simulink model "BusCreator"  (R2018b)
settings: Solver=FixedStepDiscrete  StartTime=0.0  StopTime=10.0  RelTol=1e-3
settings Model: Creator=mostafa  LastModifiedBy=mostafa
settings DataIOCC: ReturnWorkspaceOutputs=on
settings OptimizationCC: DefaultParameterBehavior=Inlined  EnhancedBackFolding=on  PassReuseOutputArgsAs=Individual arguments  ZeroExternalMemoryAtStartup=off  ZeroInternalMemoryAtStartup=off  OptimizeBlockOrder=speed  DifferentSizesBufferReuse=on  OptimizationCustomize=off
settings DebuggingCC: UnderspecifiedInitializationDetection=Classic  MergeDetectMultiDrivingBlocksExec=none  ParameterTunabilityLossMsg=error  SFMachineParentedDataDiag=error
settings ModelReferenceCC: PropagateSignalLabelsOutOfModel=off
settings SFSimCC: SimCustomHeaderCode="#include \"Interface.h\""  SimUserSources=Interface.h  MATLABDynamicMemAlloc=off
settings RTWCC: SystemTargetFile=ert.tlc  GenCodeOnly=on  TemplateMakefile=ert_default_tmf  GenerateReport=on  IncludeHyperlinkInReport=on  LaunchReport=on  GenerateTraceInfo=on  GenerateTraceReport=on  GenerateTraceReportSl=on  GenerateTraceReportSf=on  GenerateTraceReportEml=on
settings CodeAppCC: ForceParamTrailComments=on  IgnoreCustomStorageClasses=off  OperatorAnnotations=on  SimulinkDataObjDesc=on  SFDataObjDesc=on  InsertBlockDesc=on
settings ERTTargetCC: TargetLangStandard=C99 (ISO)  GenerateSampleERTMain=on  InlinedParameterPlacement=NonHierarchical  ERTCustomFileTemplate=example_file_process.tlc

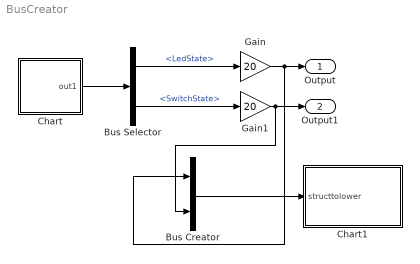
== system BusCreator ==
  Bus Creator : BusCreator  Inputs=2
  Bus Selector : BusSelector  OutputSignals=LedState,SwitchState
  Chart : Stateflow chart  TreatAsAtomicUnit=on
  Chart1 : Stateflow chart  TreatAsAtomicUnit=on
  Gain : Gain  Gain=20
  Gain1 : Gain  Gain=20
  Output : Outport
  Output1 : Outport  Port=2
  wires:
  Bus Selector/2 -> Gain1/1  "<SwitchState>"
  Bus Selector/1 -> Gain/1  "<LedState>"
  Gain/1 -> Bus Creator/1, Output/1
  Gain1/1 -> Bus Creator/2, Output1/1
  Chart/1(out1) -> Bus Selector/1
  Bus Creator/1 -> Chart1/1(structtolower)

== stateflow chart BusCreator/Chart1 ==
  (default) -> (junction 3) : {
      | setter(&structtolower);
      | }
  data: structtolower input Bus: GrOfSignals

== stateflow chart BusCreator/Chart ==
  (default) -> (junction 3) : {
      | getter(&out1);
      | }
  data: out1 output Bus: GrOfSignals
